simulink model "linsim"  (R2025a)
settings: Solver=FixedStepAuto  StartTime=0.0  StopTime=100  FixedStep=0.01  RelTol=1e-3
values from neighbouring files (symbols this model uses):
  A = [0,0,0,0,0,0,1,0,0,0,0,0 ... (first row only)    [FP_P9.m]    (also in linsim_script.m; nonlinsim_script.m; params.m)
  B = [0,0,0 ... (first row only)    [FP_P9.m]    (also in linsim_script.m; nonlinsim_script.m; params.m)
  C = Kp + Ki/s + Kd*s    [FP_P5.m]    (also in FP_P9.m = eye(12); linsim_script.m = [1,0,0,0,0,0,0,0,0,0,0,0; nonlinsim_script.m = [1,0,0,0,0,0,0,0,0,0,0,0; params.m = [1,0,0,0,0,0,0,0,0,0,0,0)
  D = zeros(12, 3)    [FP_P9.m]    (also in linsim_script.m = [0,0,0; nonlinsim_script.m = [0,0,0; params.m = [0,0,0)
  g = p(6)    [.m]    (also in FP_P9.m = 3.711; NLS_Dynamics.m; NLS_Dynamics_bonus_skycrane.m; linsim_script.m = 3.711)
  M = p(1)    [.m]    (also in FP_P9.m = 1025; NLS_Dynamics.m; NLS_Dynamics_bonus_skycrane.m; linsim_script.m = 1025)
  m = p(2)    [.m]    (also in FP_P9.m = 500; NLS_Dynamics.m; NLS_Dynamics_bonus_skycrane.m; linsim_script.m = 500)
  x0 = zeros(12,1)    [.m]    (also in FP_P9.m; NLS_Dynamics.m; NLS_Dynamics_bonus_skycrane.m; linsim_script.m)
libraries: simulink x2, slpidlib x1
settings Model: Creator=jonl6  LastModifiedBy=kritt
settings SolverCC: AlgebraicLoopSolver=TrustRegion
settings DebuggingCC: UnconnectedInputMsg=warning  UnconnectedOutputMsg=warning  UnconnectedLineMsg=warning
settings ModelReferenceCC: EnableRefExpFcnMdlSchedulingChecks=on
settings RTWCC: GPUComputeCapability=3.5

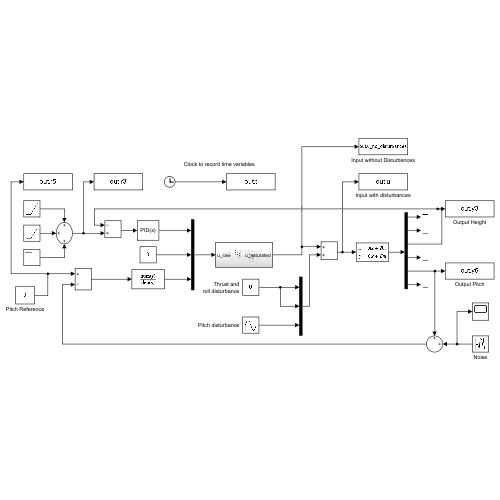
[thumbnail: Simulink's stored preview of the top-level diagram]
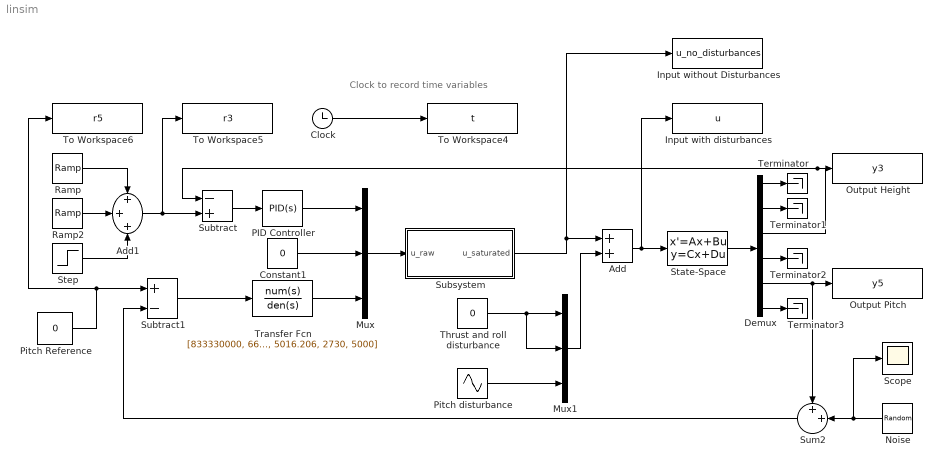
== system linsim ==
  note: Clock to record time variables
  Add : Sum
  Add1 : Sum  Inputs=+++
  Clock : Clock
  Constant1 : Constant  Value=0
  Demux : Demux  Outputs=6
  Input with disturbances : ToWorkspace  VariableName=u  SampleTime=-1
  Input without Disturbances : ToWorkspace  VariableName=u_no_disturbances  SampleTime=-1
  Mux : Mux  Inputs=3
  Mux1 : Mux  Inputs=3
  Noise : RandomNumber  Variance=1e-3  SampleTime=0.01
  Output Height : ToWorkspace  VariableName=y3  SampleTime=-1
  Output Pitch : ToWorkspace  VariableName=y5  SampleTime=-1
  PID Controller : slpidlib/PID Controller  Controller=PID  Form=Parallel  TimeDomain=Continuous-time  UseExternalTs=off  SampleTime=-1  IntegratorMethod=Forward Euler  FilterMethod=Forward Euler  ControllerParametersSource=internal  P=5000  I=0.5  UseKiTs=off  D=9000  UseExternalDerivativeSource=off  N=100  UseFilter=on  TunerSelectOption=Transfer Function Based (PID Tuner App)  InitialConditionSource=internal  InitialConditionForIntegrator=0  InitialConditionForFilter=0  DifferentiatorICPrevScaledInput=0  ExternalReset=none  TrackingMode=off  Kt=1  LimitOutput=off  SatLimitsSource=internal  UpperSaturationLimit=inf  LowerSaturationLimit=-inf  LinearizeAsGain=on  AntiWindupMode=none  Kb=1  LimitIntegrator=off  UpperIntegratorSaturationLimit=inf  LowerIntegratorSaturationLimit=-inf  POutMin=[]  POutMax=[]  IOutMin=[]  IOutMax=[]  DOutMin=[]  DOutMax=[]  NOutMin=[]  NOutMax=[]  SumOutMin=[]  SumOutMax=[]  SaturationOutMin=[]  SaturationOutMax=[]  PParamMin=[]  PParamMax=[]  IParamMin=[]  IParamMax=[]  DParamMin=[]  DParamMax=[]  NParamMin=[]  NParamMax=[]  KbParamMin=[]  KbParamMax=[]  KtParamMin=[]  KtParamMax=[]  KbOutMin=[]  KbOutMax=[]  KtOutMin=[]  KtOutMax=[]  IntegratorOutMin=[]  IntegratorOutMax=[]  FilterOutMin=[]  FilterOutMax=[]  SumI1OutMin=[]  SumI1OutMax=[]  SumI2OutMin=[]  SumI2OutMax=[]  SumI3OutMin=[]  SumI3OutMax=[]  SumI4OutMin=[]  SumI4OutMax=[]  SumDOutMin=[]  SumDOutMax=[]  DifferentiatorOutMin=[]  DifferentiatorOutMax=[]  FilterDiffOutCoefMin=[]  FilterDiffOutCoefMax=[]  ReciprocalOutMin=[]  ReciprocalOutMax=[]  SumDenOutMin=[]  SumDenOutMax=[]  SumNumOutMin=[]  SumNumOutMax=[]  DivideOutMin=[]  DivideOutMax=[]  UdiffTsProdOutMin=[]  UdiffTsProdOutMax=[]  NTsProdOutMin=[]  NTsProdOutMax=[]  UintegralTsProdOutMin=[]  UintegralTsProdOutMax=[]  UngainTsProdOutMin=[]  UngainTsProdOutMax=[]  ClampingZeroOutDataTypeStr=Inherit: Inherit via back propagation  ClampingZeroOutMin=[]  ClampingZeroOutMax=[]  FilterDenConstantOutDataTypeStr=Inherit: Inherit via back propagation  FilterDenConstantOutMin=[]  FilterDenConstantOutMax=[]  PCopyOutDataTypeStr=Inherit: Inherit via back propagation  PCopyOutMin=[]  PCopyOutMax=[]  NCopyOutDataTypeStr=Inherit: Inherit via back propagation  NCopyOutMin=[]  NCopyOutMax=[]  IntegratorContinuousStateAttributes=''  IntegratorStateMustResolveToSignalObject=off  IntegratorRTWStateStorageClass=Auto  FilterContinuousStateAttributes=''  FilterStateMustResolveToSignalObject=off  FilterRTWStateStorageClass=Auto  ParallelPVariant=InternalParameters  IdealPVariant=Disabled  IVariant=InternalParameters  DVariant=InternalParameters  IntegratorVariant=Continuous  SatVariant=Disabled  AWVariant=Passthrough  PCopyVariant=Disabled  TRVariant=Disabled  FdbkBlocksVariant=Forward  IdealPFdbkVariant=Disabled  SatFdbkVariant=Disabled  DerivativeFilterVariant=ContFilter  NVariant=InternalParameters  NCopyVariant=Disabled  FilterICVariant=InternalICsFilter  IntegratorICVariant=InternalICs  ExternalResetVariant=Disabled  TRSumVariant=Passthrough  SumFdbkVariant=Disabled  SumVariant=Sum_PID  TsampFilterVariant=InternalTs  TsampNgainVariant=Passthrough  TsampIntegralVariant=Disabled_SignalSpec  ExternalSaturationOutDataTypeStr=Inherit: Same as second input  DerivativeSourceVariant=ErrorSignal  PreIntVariant=InternalPreInt
  Pitch Reference : Constant  Value=0  SampleTime=0.01
  Pitch disturbance : Sin  Amplitude=1e3  SampleTime=0
  Ramp : simulink/Sources/Ramp  slope=0.5  start=0  InitialOutput=0
  Ramp2 : simulink/Sources/Ramp  slope=-0.5  start=40  InitialOutput=0
  Scope : Scope
      settings: ActiveDisplayYMinimum=-0.11487633319149182  ActiveDisplayYMaximum=0.1254432823941159
  State-Space : StateSpace  A=A  B=B  C=C  D=D  InitialCondition=x0
  Step : Step  Time=40  After=-10  SampleTime=0
  Subsystem : Subsystem
  Subtract : Sum  Inputs=-+
  Subtract1 : Sum  Inputs=+-
  Sum2 : Sum  Inputs=++|
  Terminator{,1..3} (4 alike) : Terminator
  Thrust and roll disturbance : Constant  Value=0
  To Workspace4 : ToWorkspace  VariableName=t  SampleTime=-1
  To Workspace5 : ToWorkspace  VariableName=r3  SampleTime=-1
  To Workspace6 : ToWorkspace  VariableName=r5  SampleTime=-1
  Transfer Fcn : TransferFcn  Numerator=[833330000, 666664000, 158332700, 9999960]  Denominator=[1, 102.006, 2700.612, 5016.206, 2730, 5000]
  wires:
  State-Space/1 -> Demux/1
  Clock/1 -> To Workspace4/1
  Noise/1 -> Sum2/2, Scope/1
  Demux/3 -> Subtract/1, Output Height/1
  Add/1 -> State-Space/1, Input with disturbances/1
  Mux1/1 -> Add/2
  Demux/5 -> Output Pitch/1, Sum2/1
  Pitch disturbance/1 -> Mux1/3
  Thrust and roll disturbance/1 -> Mux1/2, Mux1/1
  Mux/1 -> Subsystem/1(u_raw)
  Subsystem/1(u_saturated) -> Add/1, Input without Disturbances/1
  Sum2/1 -> Subtract1/2
  Constant1/1 -> Mux/2
  Ramp/1 -> Add1/1
  Ramp2/1 -> Add1/2
  Step/1 -> Add1/3
  Add1/1 -> Subtract/2, To Workspace5/1
  Pitch Reference/1 -> To Workspace6/1, Subtract1/1
  PID Controller/1 -> Mux/1
  Subtract/1 -> PID Controller/1
  Subtract1/1 -> Transfer Fcn/1
  Transfer Fcn/1 -> Mux/3
  Demux/2 -> Terminator1/1
  Demux/1 -> Terminator/1
  Demux/4 -> Terminator2/1
  Demux/6 -> Terminator3/1

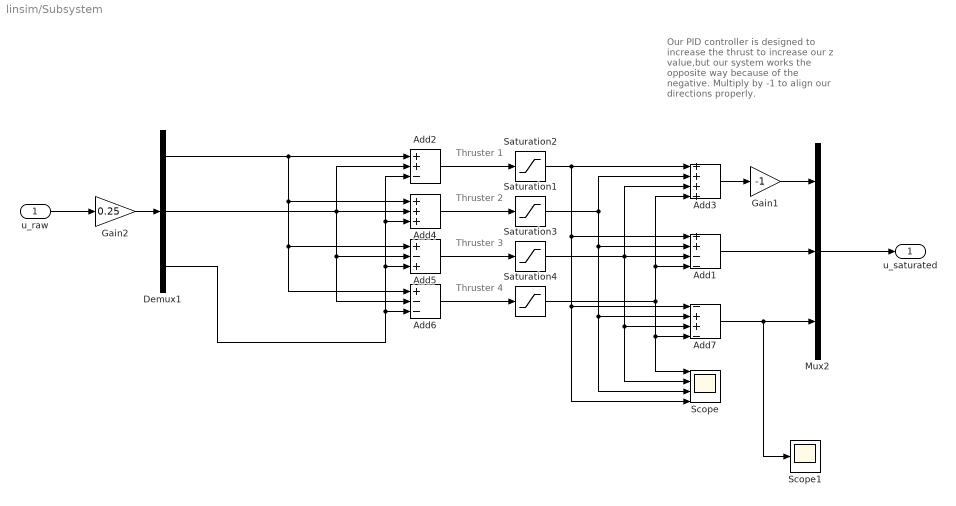
== system linsim/Subsystem ==
  note: Thruster 1
  note: Our PID controller is designed to increase the thrust to increase our z value,but our system works the opposite way because of the negative. Multiply by -1 to align our directions properly.
  note: Thruster 2
  note: Thruster 3
  note: Thruster 4
  u_raw : Inport
  Add1 : Sum  Inputs=++--
  Add2 : Sum  Inputs=++-
  Add3 : Sum  Inputs=++++
  Add4 : Sum  Inputs=+++
  Add5 : Sum  Inputs=+-+
  Add6 : Sum  Inputs=+--
  Add7 : Sum  Inputs=-++-
  Demux1 : Demux  Outputs=3
  Gain1 : Gain  Gain=-1
  Gain2 : Gain  Gain=0.25
  Mux2 : Mux  Inputs=3
  Saturation{1..4} (4 alike) : Saturate  UpperLimit=(M+m)*g  LowerLimit=-(M+m)*g/4
  Scope : Scope  NumInputPorts=4
      settings: ActiveDisplayYMinimum=-2299.08046875  ActiveDisplayYMaximum=6543.53671875  DataLoggingVariableName=ScopeData3
  Scope1 : Scope
      settings: ActiveDisplayYMinimum=-2529.571482035929  ActiveDisplayYMaximum=1070.4285179640719  DataLoggingVariableName=ScopeData9
  u_saturated : Outport
  wires:
  Add6/1 -> Saturation4/1
  Gain2/1 -> Demux1/1
  Saturation3/1 -> Scope/2, Add7/3, Add1/3, Add3/3
  Demux1/2 -> Add2/2, Add5/2, Add6/2, Add4/2
  Add1/1 -> Mux2/2
  Add4/1 -> Saturation1/1
  Saturation4/1 -> Scope/1, Add7/4, Add1/4, Add3/4
  Demux1/3 -> Add2/3, Add4/3, Add5/3, Add6/3
  Add2/1 -> Saturation2/1
  Saturation1/1 -> Scope/3, Add7/2, Add1/2, Add3/2
  u_raw/1 -> Gain2/1
  Add5/1 -> Saturation3/1
  Add7/1 -> Scope1/1, Mux2/3
  Mux2/1 -> u_saturated/1
  Demux1/1 -> Add2/1, Add4/1, Add5/1, Add6/1
  Add3/1 -> Gain1/1
  Saturation2/1 -> Add3/1, Scope/4, Add7/1, Add1/1
  Gain1/1 -> Mux2/1
